simulink library "MCHP_Blockset"  (R2014b)
settings: Solver=ode45  SolverMode=SingleTasking  StartTime=0.0  StopTime=10.0  RelTol=1e-3
InitFcn:
  | disp('MCHP_Blockset_Library_InitFunction');
undefined symbols (not defined in the file): A0, A2, AD0, AVdd, B1, B5, B9, C10, C2, CMP2A, CMP3A, CMP4A, EXTREF1, EXTREF2, gcbh, MaxPer, MCHP_ACC_SAMx_Callback, MCHP_ADC_Callback, MCHP_ADC_HighSpeed_SAR_Callback, MCHP_ADC_HighSpeed_SAR_dsPIC_Callback, MCHP_ADC_SAME5x_Callback, MCHP_AFEC_SAM7x_Callback, MCHP_BUS_I2C_MASTER_callback, MCHP_BUS_SPI_callback, MCHP_C_function_Call_callback, MCHP_CN_Callback, MCHP_COMPARATOR1_callback, MCHP_CompilerOptimisation_Callback, MCHP_DACC_SAMx_Callback, MCHP_Digital_Input_Callback, MCHP_Digital_Output_Read_Callback, MCHP_Digital_Output_Write_Callback, MCHP_Fun, MCHP_HighSpeed_AnalogComparator_Callback, MCHP_IC_Callback, MCHP_IdleTask_Callback, MCHP_Interrupt_Callback, MCHP_Master_Callback, MCHP_MCPWM_Callback, MCHP_MCU_LOAD_Callback, MCHP_MCU_OVERLOAD_Callback, MCHP_MSI_Callback, MCHP_OC_HW_Callback, MCHP_OC_SW_Callback, MCHP_OP_AMP_Callback, MCHP_OrderInOut, MCHP_PDEC_Callback, MCHP_PGA_Callback, MCHP_PWM_Callback, MCHP_PWM_HighSpeed_Override_Callback, MCHP_PWM_HS_FEP_Callback, MCHP_PWM_SAM7x_Callback, MCHP_PWM_SAM7x_Override_Callback, MCHP_QDEC_SAMx_Callback, MCHP_QEI_Callback, MCHP_Scheduler_Options_Callback, MCHP_SECONDARY_CORE_Callback, MCHP_Tasks_State_Callback, MCHP_TCC_PWM_Callback, MCHP_TIMER_Config_Callback ... (+18)
libraries: MCHP_Blockset x2
(part 4 of 9)

== system MCHP_Blockset/BUS I2C ==
  BUS I2C MASTER : S-Function  FunctionName=MCHP_BUS_I2C_MASTER  Parameters=MCHP_BUS_I2C_MASTER_callback(gcbh,'S_INPUT'),MCHP_BUS_I2C_MASTER_callback(gcbh,'S_OUTPUT'),MCHP_BUS_I2C_MASTER_callback(gcbh,'S_INPUT_Size'),MCHP_BUS_I2C_MASTER_callback(gcbh,'S_OUTPUT_Size'),[],SampleTime,MCHP_OrderInOut(gcbh),strcmp(BlockingMode,'on')  EnableBusSupport=off  mask(I2C Driver){I2CRef=1, I2C_IntPriority=5, I2Csequence_txt=Initial-Configuration$     ---     $Start$Write Address:{[0x77]}    % Componnent address$Write Data (x1)  Write:{[0x00]}      % Write a constant$Re-Start$Read Data (x1)  Read:{D2}    % Read a value$Stop, I2Csequence_num=[BFF0000000000000 40E0600000000000 40F86A0000000000 40F866E066594CA2]$[4070000000000000]$[3FF0000000000000 40E0200000000000 40F86A0000000000 40F866E066594CA2]$[4040000000000000 0000000000000000 0000000000000000 405DC00000000000]$[4050000000000000 3FF0000000000000 0000000000000000 0000000000000000]$[4008000000000000 40E0200000000000 40F86A0000000000 40F866E066594CA2]$[4060000000000000 3FF0000000000000]$[4000000000000000 40E0600000000000 40F86A0000000000 40F866E066594CA2], InitialConfigurationNum=0, PIN_SDA_TXT=Dynamic Options, PIN_SCL_TXT=Dynamic Options, S_INPUT=[5  5], S_OUTPUT=[5], S_INPUT_Size=[2  2], S_OUTPUT_Size=[4], BlockingMode=off, SequenceCompleted=off, SampleTime=-1, MCHP_MASTERLINK=Board28PIN_33EP12MC202_I2C_MS5611_V02/Microchip Master, MCHP_PORT={I2C 1 Clock}{SCL1}13:0:B8;{I2C 1 SDA}{SDA1}13:0:B9;, MCHP_USER_INTERRUPTS=, ORDERING=0}
      mask prompts: I2C_IntPriority "Interrupt Priority"; I2Csequence_txt "I2C_Sequence"; I2Csequence_num "I2C_Sequence"; SampleTime "Sample Time"; ORDERING "MCHP_OrderInOut"
      mask init:
      | MCHP_BUS_I2C_MASTER_callback(gcbh,'INITIALISATION');
      settings: CopyFcn=MCHP_BUS_I2C_MASTER_callback(gcbh,'COPY');  DeleteFcn=MCHP_BUS_I2C_MASTER_callback(gcbh,'DELETE');  ModelCloseFcn=MCHP_BUS_I2C_MASTER_callback(gcbh,'MODELCLOSE');  OpenFcn=MCHP_BUS_I2C_MASTER_callback(gcbh,'OPEN');
      mask Display:
      | MCHP_DrawLogo;fprintf(['I2C ' int2str(I2CRef) ' ']);
      | 
      | port_label('output',1,'1/z*D2');

== system MCHP_Blockset/BUS SPI ==
  BUS SPI : S-Function  FunctionName=MCHP_BUS_SPI  Parameters=MCHP_BUS_SPI_callback(gcbh,'S_INPUT'),MCHP_BUS_SPI_callback(gcbh,'S_OUTPUT'),MCHP_BUS_SPI_callback(gcbh,'S_INPUT_Size'),MCHP_BUS_SPI_callback(gcbh,'S_OUTPUT_Size'),[],SampleTime,MCHP_OrderInOut(gcbh),strcmp(BlockingMode,'on')  EnableBusSupport=off  mask(SPI Driver){SPIRef=1, DMA=[0  2  3], SPI_IntPriority=4, SPIsequence_txt=Initial-Configuration$     ---     $Set Port B6 / Pin[42] to 1$Read & Write (x1)  Write:{In}  Read:{out}$Set Port B6 / Pin[42] to 0, SPIsequence_num=[BFF0000000000000 4091B40000000000 0000000000000000 40E0000000000000 411E848000000000 411E848000000000]$[4070000000000000]$[4010000000000000 4036000000000000 3FF0000000000000]$[4008000000000000 3FF0000000000000 3FF0000000000000]$[4010000000000000 4036000000000000 0000000000000000], PIN_SDI_TXT=Dynamic Options, PIN_SDO_TXT=Dynamic Options, PIN_SCK_TXT=Dynamic Options, PIN_SS_TXT=Dynamic Options, S_INPUT=[5  5], S_OUTPUT=[5], S_INPUT_Size=[2  2], S_OUTPUT_Size=[4], BlockingMode=off, SampleTime=-1, MCHP_MASTERLINK=UTester_33EP64MC504_SPI/Microchip Master, MCHP_PORT={SPI 1 input}{SDI1}12:0:A9;{SPI 1 output}{SDO1}12:1:A4;{SPI 1 Clock output}{SCK1}12:1:C3;{SPI 1 PIN output}{SPI1 Pin}12:1:B6;{SPI 1 PIN output}{SPI1 Pin}12:1:B6;, MCHP_USER_INTERRUPTS=, ORDERING=0}
      mask prompts: DMA "DMA [Enabled(0/1) Rx Tx]"; SPI_IntPriority "Interrupt Priority"; SPIsequence_txt "SPI_Sequence"; SPIsequence_num "SPI_Sequence"; SampleTime "Sample Time"; ORDERING "MCHP_OrderInOut"
      mask init:
      | MCHP_BUS_SPI_callback(gcbh,'INITIALISATION');
      settings: CopyFcn=MCHP_BUS_SPI_callback(gcbh,'COPY');  DeleteFcn=MCHP_BUS_SPI_callback(gcbh,'DELETE');  ModelCloseFcn=MCHP_BUS_SPI_callback(gcbh,'MODELCLOSE');  OpenFcn=MCHP_BUS_SPI_callback(gcbh,'OPEN');
      mask Display:
      | MCHP_DrawLogo;fprintf(['SPI ' int2str(SPIRef) ' ']);
      | 
      | port_label('input',1,'In');
      | port_label('output',1,'1/z*out');

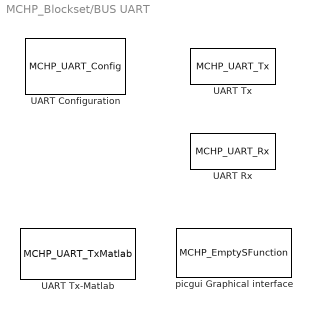
== system MCHP_Blockset/BUS UART ==
  UART Configuration : S-Function  InitFcn=MCHP_UART_Config_Callback(gcbh,'InitFcn');  FunctionName=MCHP_UART_Config  EnableBusSupport=off  mask(Configuration for UART peripheral){UART_REF=1, BAUD_Choice=Dynamic Options, BAUD_Choice_TXT=115200, BAUD_Choice_IR=Dynamic Options, BAUD_Choice_IR_TXT=[], BAUD_Custom=115200, INT_PRIORITY=0, ALT_IO=on, PIN_RX=Dynamic Options, PIN_RX_TXT=Dynamic Options, PIN_TX=Dynamic Options, PIN_TX_TXT=Dynamic Options, MCHP_PORT={UART1  Rx}{U1RX}3:0:P25;{UART1  Tx}{U1TX}3:1:P20;, MCHP_MASTERLINK=0, MCHP_COM_ExtPil=off, TX_IMPLEMENTATION=Circular Buffer, TX_IMPLEMENTATION_default=Circular Buffer, TX_INT_PRIORITY=5, TX_INT_WHEN=is empty, TX_INT_WHEN_default=is empty & last char is sent, TX_CIRCULAR_SIZE=128, TX_DMA_CHANNEL=0   (Lowest Priority), TX_DMA_SIZE=[], TX_TASK_PROTECTION=Delay tasks (default), TX_INTERRUPT_PROTECTION=Do not send on conflict (default), TX_INTERRUPT_PROTECTION_default=Do not send on conflict (default), RX_IMPLEMENTATION=Circular Buffer, RX_IMPLEMENTATION_default=Circular Buffer, RX_INT_PRIORITY=5, RX_INT_WHEN=receive 1 character, RX_CIRCULAR_SIZE=128, RX_DMA_CHANNEL=0, RX_DMA_SIZE=0, DuplexMode=Full duplex (default), PIN_RX_Inv=off, PIN_TX_Inv=off, PIN_RXTX_Inv=off, ParityBit=No parity (default), StopBit=1 stop bit (default), IRDA=off, FlowControl=None, PIN_CTS=Dynamic Options, PIN_CTS_TXT=Dynamic Options, PIN_RTS=Dynamic Options, PIN_RTS_TXT=Dynamic Options, InitSequence_chkbox=off, BAUD_Choice_InitSeq=Dynamic Options, BAUD_Choice_InitSeq_TXT=0, BAUD_Choice_IR_InitSeq=Dynamic Options, BAUD_Choice_IR_InitSeq_TXT=0, BAUD_Custom_InitSeq=0, InitSequence='Hello World'}
      mask prompts: UART_REF "Ref UART"; BAUD_Choice "Current Baud:"; BAUD_Choice_TXT "Baud_Choixe_TXT"; BAUD_Choice_IR "Current Baud:"; BAUD_Custom "Custom Baud: 109306 with -5.12% Error"; INT_PRIORITY "Interrupt Priority"; ALT_IO "Alternative I/O"; PIN_RX "Rx Pin"; PIN_TX "Tx Pin"; TX_IMPLEMENTATION "Implementation"; TX_IMPLEMENTATION_default "Implementation"; TX_INT_PRIORITY "Interrupt Priority"; TX_INT_WHEN "Interrupt when Transmit Buffer"; TX_INT_WHEN_default "Interrupt when Transmit Buffer"; TX_CIRCULAR_SIZE "Circular Buffer size"; TX_DMA_CHANNEL "DMA Channel"; TX_DMA_SIZE "DMA Buffer size"; TX_TASK_PROTECTION "Task intertwined Tx protection"; TX_INTERRUPT_PROTECTION "Asynchronous intertwined Tx protection"; TX_INTERRUPT_PROTECTION_default "Asynchronous intertwined Tx protection"; RX_IMPLEMENTATION "Implementation"; RX_IMPLEMENTATION_default "Implementation"; RX_INT_PRIORITY "Interrupt Priority"; RX_INT_WHEN "Interrupt when Receive Buffer"; RX_CIRCULAR_SIZE "Circular Buffer size"; RX_DMA_CHANNEL "DMA Channel"; RX_DMA_SIZE "DMA Buffer size"; DuplexMode "Duplex"; PIN_RX_Inv "Invert Rx Pin logic (Idle state is low level)"; PIN_TX_Inv "Invert Tx Pin logic (Idle state is low level)"; PIN_RXTX_Inv "Invert Rx & Tx Pin logic (Idle state is low level)"; ParityBit "Parity"; StopBit "Stop bit"; IRDA "IrDA Mode"; FlowControl "Hardware Flow Control"; PIN_CTS "CTS Pin (input)"; PIN_RTS "RTS Pin (output)"; InitSequence_chkbox "Send an Initialisation sequence on the UART"; BAUD_Choice_InitSeq "Baud for initialisation sequence:"; BAUD_Choice_InitSeq_TXT "Baud_Choixe_TXT"; BAUD_Choice_IR_InitSeq "Baud for initialisation sequence:"; BAUD_Choice_IR_InitSeq_TXT "Baud_Choice_IR_TXT"; BAUD_Custom_InitSeq "Custom Baud: 109306 with -5.12% Error"; InitSequence "Initialisaiton sequence to send (String or vector)"
      mask init:
      | MCHP_UART_Config_Callback(gcbh,'INITIALISATION');
      settings: CopyFcn=MCHP_UART_Config_Callback(gcbh,'CopyFcn');  PreSaveFcn=MCHP_Fun.PreSaveFcn_DynamicOptions(gcbh);  OpenFcn=MCHP_UART_Config_Callback(gcbh,'OPEN');
      mask TypeOptions UART_REF: 1 | 2 | 3 | 4 | 5 | 6 | 7 | 8 | 9 | USART 0 | USART 1 | USART 2 | USART 3 | USART 4 | USART 5 | USART 6 | USART 7 | USART 8 | ----------- | UART 0 | UART 1 | UART 2 | UART 3 | UART 4 | UART 5 | UART 6 | UART 7 | UART 8 | --SAMx5----- | SERCOM USART 0 | SERCOM USART 1 | SERCOM USART 2 | SERCOM USART 3 | SERCOM USART 4 | SERCOM USART 5 | SERCOM USART 6 | SERCOM USART 7 | SERCOM USART 8 | SERCOM USART 9
      mask Callback UART_REF: MCHP_UART_Config_Callback(gcbh,'UART_REF');
      mask TypeOptions BAUD_Choice: Dynamic Options
      mask Callback BAUD_Choice: MCHP_UART_Config_Callback(gcbh,'BAUD_Choice');
      mask TypeOptions BAUD_Choice_IR: Dynamic Options
      mask Callback BAUD_Choice_IR: MCHP_UART_Config_Callback(gcbh,'BAUD_Choice_IR');
      mask Callback BAUD_Choice_IR_TXT: % This field is not used
      mask Callback BAUD_Custom: MCHP_UART_Config_Callback(gcbh,'BAUD_Custom');
      mask TypeOptions INT_PRIORITY: 0 | 1 | 2 | 3 | 4 | 5 | 6 | 7
      mask TypeOptions PIN_RX: Dynamic Options
      mask TypeOptions PIN_TX: Dynamic Options
      mask TypeOptions TX_IMPLEMENTATION: Do not implement Tx | Simplest (1 bytes internal buffer only) | Simplest (4 bytes internal buffer only) | Simplest (8 bytes internal buffer only) | Circular Buffer | DMA Ping-Pong Mode | DMA single Buffer (Possible data loss)
      mask Callback TX_IMPLEMENTATION: MCHP_UART_Config_Callback(gcbh,'TX_IMPLEMENTATION');
      mask TypeOptions TX_IMPLEMENTATION_default: Circular Buffer
      mask TypeOptions TX_INT_PRIORITY: 0 | 1 | 2 | 3 | 4 | 5 | 6 | 7
      mask TypeOptions TX_INT_WHEN: is empty | is empty & last char is sent | has one empty space
      mask TypeOptions TX_INT_WHEN_default: is empty & last char is sent
      mask TypeOptions TX_CIRCULAR_SIZE: 4 | 8 | 16 | 32 | 64 | 128 | 256 | 512 | 1024 | 2048 | 4096 | 8192 | 16384 | 32768
      mask TypeOptions TX_DMA_CHANNEL: 0 | 0   (Lowest Priority) | 1 | 2 | 3 | 4 | 5 | 6 | 7 | 8 | 9 | 10 | 11 | 12 | 13 | 14 | 15 | 16 | 17 | 18 | 19 | 20 | 21 | 22 | 23
      mask TypeOptions TX_TASK_PROTECTION: Delay tasks (default) | Do not send on conflict | no protection
      mask Callback TX_TASK_PROTECTION: MCHP_UART_Config_Callback(gcbh,'TX_TASK_PROTECTION');
      mask TypeOptions TX_INTERRUPT_PROTECTION: Do not send on conflict (default) | Delay all interrupts | no protection
      mask TypeOptions TX_INTERRUPT_PROTECTION_default: Do not send on conflict (default)
      mask TypeOptions RX_IMPLEMENTATION: Do not implement Rx | Simplest (1 bytes internal buffer only) | Simplest (4 bytes internal buffer only) | Simplest (8 bytes internal buffer only) | Circular Buffer | DMA Ping-Pong | DMA Single Buffer (possible data loss)
      mask Callback RX_IMPLEMENTATION: MCHP_UART_Config_Callback(gcbh,'RX_IMPLEMENTATION');
      mask TypeOptions RX_IMPLEMENTATION_default: Circular Buffer
      mask TypeOptions RX_INT_PRIORITY: 1 | 2 | 3 | 4 | 5 | 6 | 7
      mask TypeOptions RX_INT_WHEN: is full (contains 4 data characters) | is 3/4 fulll (contains 3 data characters) | receive 1 character
      mask TypeOptions RX_CIRCULAR_SIZE: 4 | 8 | 16 | 32 | 64 | 128 | 256 | 512 | 1024 | 2048 | 4096 | 8192 | 16384 | 32768
      mask TypeOptions RX_DMA_CHANNEL: 0 | 0   (Lowest Priority) | 1 | 2 | 3 | 4 | 5 | 6 | 7 | 8 | 9 | 10 | 11 | 12 | 13 | 14 | 15 | 16 | 17 | 18 | 19 | 20 | 21 | 22 | 23
      mask TypeOptions DuplexMode: Full duplex (default) | Half duplex for one wire Rx-Tx specific case
      mask Callback DuplexMode: MCHP_UART_Config_Callback(gcbh,'DuplexMode');
      mask TypeOptions ParityBit: No parity (default) | Even | Odd | Space (force to 0) | Mark (force to 1) | Multidrop
      mask TypeOptions StopBit: 1 stop bit (default) | 1.5 stop bits | 2 stop bits
      mask Callback IRDA: MCHP_UART_Config_Callback(gcbh,'IRDA');
      mask TypeOptions FlowControl: None | RTS / CTS
      mask Callback FlowControl: MCHP_UART_Config_Callback(gcbh,'FlowControl');
      mask TypeOptions PIN_CTS: Dynamic Options
      mask TypeOptions PIN_RTS: Dynamic Options
      mask Callback InitSequence_chkbox: MCHP_UART_Config_Callback(gcbh,'InitSequence_chkbox');
      mask TypeOptions BAUD_Choice_InitSeq: Dynamic Options
      mask Callback BAUD_Choice_InitSeq: MCHP_UART_Config_Callback(gcbh,'BAUD_Choice_InitSeq');
      mask TypeOptions BAUD_Choice_IR_InitSeq: Dynamic Options
      mask Callback BAUD_Choice_IR_InitSeq: MCHP_UART_Config_Callback(gcbh,'BAUD_Choice_IR_InitSeq');
      mask Callback BAUD_Custom_InitSeq: MCHP_UART_Config_Callback(gcbh,'BAUD_Custom_InitSeq');
      mask Display:
      | MCHP_DrawLogo;
      | disp('UART Config');
  UART Rx : S-Function  FunctionName=MCHP_UART_Rx  Parameters=SampleTime,strcmp(Flag_Out,'on'),S_Rx_Size,MCHP_OrderInOut(gcbh)  EnableBusSupport=off  mask(UART Rx Input Driver){UART_REF=1, Flag_Out=off, Rx_Size_popup=User defined, Rx_Size=1, S_Rx_Size=1, Split=Read all received char, SplitChar=10, OutputDefault_popup=Fill-in output vector with specified value, OutputDefault=-1, ORDERING=None, SampleTime=-1, MCHP_MASTERLINK=UTestBoard_33FJ256GP710A_2/Microchip Master, MCHP_COMPILED_INFO=0}
      mask prompts: UART_REF "UART Ref"; Flag_Out "Output Number of char read"; Rx_Size_popup "Vector Output size"; Rx_Size "Vector Output size (i.e. try to read n char)"; SplitChar "Stop reading on character: (split)"; OutputDefault_popup "Fill-in output vector when not full:"; OutputDefault "Output Vector not full: fill in with value: (-1 repeat last char, -2: do nothing)"; ORDERING "Block execution ordering"; SampleTime "Sample Time"
      mask help:
      | Receive data (8 bits datatype) through the UART.use >>picgui at the Matlab prompt in "raw" mode to send/receive data with matlab.
      |
      | UART Ports: [ Rx  Tx  ]
      | UART 1:         [ F2  F3 ]
      | UART 2:         [ F4  F5 ]
      |
      | UART 2 is configured at:   115200         [-0.04%]
      mask init:
      | MCHP_UART_Rx_Callback(gcbh,'INITIALISATION');
      settings: OpenFcn=MCHP_UART_Rx_Callback(gcbh,'OPEN');
      mask TypeOptions UART_REF: 1 | 2 | 3 | 4 | 5 | 6 | 7 | 8 | 9 | USART 0 | USART 1 | USART 2 | USART 3 | USART 4 | USART 5 | USART 6 | USART 7 | USART 8 | ----------- | UART 0 | UART 1 | UART 2 | UART 3 | UART 4 | UART 5 | UART 6 | UART 7 | UART 8
      mask Callback UART_REF: MCHP_UART_Rx_Callback(gcbh,'UART_REF');
      mask TypeOptions Rx_Size_popup: User defined | Inherited via back propagation | Inherited via internal rule
      mask Callback Rx_Size_popup: MCHP_UART_Rx_Callback(gcbh,'Rx_Size_popup');
      mask Callback Rx_Size: MCHP_UART_Rx_Callback(gcbh,'Rx_Size');
      mask TypeOptions Split: Read all received char | Stop reading when one specified char is detected
      mask Callback Split: MCHP_UART_Rx_Callback(gcbh,'Split');
      mask TypeOptions OutputDefault_popup: Fill-in output vector with specified value | Add one trailing 0 | do nothing (end of output vector will be undefined)
      mask Callback OutputDefault_popup: MCHP_UART_Rx_Callback(gcbh,'OutputDefault_popup');
      mask TypeOptions ORDERING: None | Input | Output | Input & Output
      mask Display: MCHP_DrawLogo;fprintf('UART 1\nRx');port_label('output',1,'Rx' );
  UART Tx : S-Function  FunctionName=MCHP_UART_Tx  Parameters=SampleTime,MCHP_OrderInOut(gcbh),NSend_Input,NSend_Output  EnableBusSupport=off  mask(UART Tx Output Driver){UART_REF=1, ORDERING=None, AllOrNothing=off, SampleTime=-1, MCHP_MASTERLINK=0, NSend_Input=off, UART_String=off, NSend_Output=off}
      mask prompts: UART_REF "UART Ref"; ORDERING "Block execution ordering"; AllOrNothing "UART Overflow: Send all or nothing"; SampleTime "Sample Time"; NSend_Input "Send first N bytes from the vector input with N a block input"; UART_String "With vector input, do not send values following the first 0 (string like)"; NSend_Output "Number of byte sent is a block output"
      mask init:
      | MCHP_UART_Tx_Callback(gcbh,'INITIALISATION');
      settings: OpenFcn=MCHP_UART_Tx_Callback(gcbh,'OPEN');
      mask TypeOptions UART_REF: 0 | 1 | 2 | 3 | 4 | 5 | 6 | 7 | 8 | 9 | USART 0 | USART 1 | USART 2 | USART 3 | USART 4 | USART 5 | USART 6 | USART 7 | USART 8 | ----------- | UART 0 | UART 1 | UART 2 | UART 3 | UART 4 | UART 5 | UART 6 | UART 7 | UART 8
      mask Callback UART_REF: MCHP_UART_Tx_Callback(gcbh,'UART_REF');
      mask TypeOptions ORDERING: None | Input | Output | Input & Output
      mask Display: MCHP_DrawLogo;fprintf('UART 1\nTx');port_label('input',1,'Tx' );
  UART Tx-Matlab : S-Function  FunctionName=MCHP_UART_TxMatlab  Parameters=SampleTime,MCHP_UART_TxMatlab_Callback(gcbh,'S_INPUT')  EnableBusSupport=off  mask(Higl Level UART protocol){UART_REF=1, CHANNELS=[1 2 ], AllOrNothing=off, SampleTime=-1, MCHP_MASTERLINK=MCHP_Blockset/System Configuration/Microchip Master, MCHP_COMPILED_INFO=CompiledSampleTime= [0.001   0 ];CompiledPortDataTypes=[  5   5   5   5   5   3 ];}
      mask prompts: UART_REF "UART Ref"; CHANNELS "Channels (Matlab Columns)"; AllOrNothing "UART Overflow: Send all or nothing"; SampleTime "Sample Time"
      mask init:
      | MCHP_UART_TxMatlab_Callback(gcbh,'INITIALISATION');
      settings: OpenFcn=MCHP_UART_TxMatlab_Callback(gcbh,'OPEN');
      mask TypeOptions UART_REF: 0 | 1 | 2 | 3 | 4 | 5 | 6 | 7 | 8 | 9 | USART 0 | USART 1 | USART 2 | USART 3 | USART 4 | USART 5 | USART 6 | USART 7 | USART 8 | ----------- | UART 0 | UART 1 | UART 2 | UART 3 | UART 4 | UART 5 | UART 6 | UART 7 | UART 8
      mask Callback UART_REF: MCHP_UART_TxMatlab_Callback(gcbh,'UART_REF');
      mask Callback CHANNELS: MCHP_UART_TxMatlab_Callback(gcbh,'INITIALISATION');
      mask Display: MCHP_DrawLogo;fprintf('UART 1\n>Matlab');port_label('input',1,'CH 1 ' );port_label('input',2,'CH 2 ' );
  picgui Graphical interface : S-Function  FunctionName=MCHP_EmptySFunction  EnableBusSupport=off  mask{Nothing=0}
      settings: OpenFcn=picgui;
      mask Display:
      | MCHP_DrawLogo;
      | color('black');
      | disp('Interface\nTx-Matlab\n>>picgui')

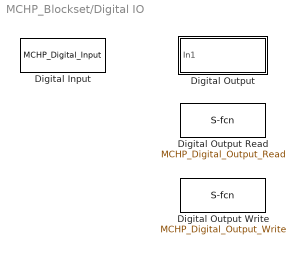
== system MCHP_Blockset/Digital IO ==
  Digital Input : S-Function  FunctionName=MCHP_Digital_Input  Parameters=SampleTime,[],MCHP_Digital_Input_Callback(gcb,'S_OUTPUT'),MCHP_OrderInOut(gcbh)  EnableBusSupport=off  mask(Input driver for Digital Input Pins){PORT=Dynamic Options, PORT_TXT=A0, PIN=[0], PACK=off, SIMULTANEOUS=off, ORDERING=None, SampleTime=-1, MCHP_PORT={Digital In}2:0:A0;, MCHP_MASTERLINK=0}
      mask prompts: PORT_TXT "Port TXT"; PIN "Pins : [ 0 : 4 ]"; PACK "set output as one uint16"; SIMULTANEOUS "Exact simultaneous sample"; ORDERING "Block execution ordering"; SampleTime "Sample Time"
      mask help:
      | Selected pin(s) are configured as a digital input.
      |
      | When the block output is defined as one uint16, user should
      | take into account only bits corresponding to pins selected.
      mask init:
      | MCHP_Digital_Input_Callback(gcb,'INITIALISATION');
      settings: PreSaveFcn=MCHP_Fun.PreSaveFcn_DynamicOptions(gcbh);  OpenFcn=MCHP_Digital_Input_Callback(gcb,'OPEN');
      mask TypeOptions PORT: Dynamic Options
      mask Callback PORT: MCHP_Fun.BlockUpdate(gcbh);
      mask Callback PIN: MCHP_Fun.BlockUpdate(gcbh);
      mask Callback PACK: MCHP_Fun.BlockUpdate(gcbh);
      mask Callback SIMULTANEOUS: %MCHP_Fun.BlockUpdate(gcbh);
      mask TypeOptions ORDERING: None | Input | Output | Input & Output
      mask Display:
      | MCHP_DrawLogo;
      | fprintf('Digital\nInput');
      | port_label('output',1,'A0');
  Digital Output : Subsystem  mask{PORT=Dynamic Options, PORT_TXT=A   [ 0  1  2  3  4  5  6  7  9  10  14  15 ], PIN=[0], PACK=off, SIMULTANEOUS=off, READPREVIOUS=off, ORDERING=None, SampleTime=-1, MCHP_PORT={Digital Out}{DOU}1:1:A0;{Digital Out}{DOU}1:1:A1;{Digital Out}{DOU}1:1:A2;, MCHP_MASTERLINK=UTester_33EP512MU810_NewDigitOutBlock/Microchip Master}
      mask prompts: PORT_TXT "Port TXT"; PIN "PORT A Indexes within [ 0  1  2  3  4  5  6  7  9  10  14  15 ]"; PACK "set input as one uint16"; SIMULTANEOUS "Exact simulatneous update"; READPREVIOUS "Read previous value written (1/z delay)"; ORDERING "Block execution ordering"; SampleTime "Sample Time"
      mask init:
      | MCHP_Digital_Output_Callback(gcb,'INITIALISATION');
      settings: PreSaveFcn=MCHP_Fun.PreSaveFcn_DynamicOptions(gcbh);  OpenFcn=MCHP_Digital_Output_Callback(gcb,'OPEN');
      mask TypeOptions PORT: Dynamic Options
      mask Callback PORT: MCHP_Fun.BlockUpdate(gcbh);
      mask Callback PIN: MCHP_Fun.BlockUpdate(gcbh);
      mask Callback PACK: MCHP_Fun.BlockUpdate(gcbh);
      mask Callback SIMULTANEOUS: MCHP_Fun.BlockUpdate(gcbh);
      mask Callback READPREVIOUS: MCHP_Fun.BlockUpdate(gcbh);
      mask TypeOptions ORDERING: None | Input | Output | Input & Output
      mask Callback ORDERING: MCHP_Fun.BlockUpdate(gcbh);
      mask Display:
      | MCHP_DrawLogo;fprintf('Digital\nOutput')
      | port_label('input',1,'A0');
  Digital Output Read : S-Function  FunctionName=MCHP_Digital_Output_Read  Parameters=SampleTime,MCHP_Digital_Output_Read_Callback(gcb,'S_INPUT'),MCHP_Digital_Output_Read_Callback(gcb,'S_OUTPUT'),MCHP_OrderInOut(gcbh)  EnableBusSupport=off  mask(Output driver for Digital Output Pins){PORT=Dynamic Options, PORT_TXT=A   [ 0  1  2  3  4  5  6  7  9  10  14  15 ], PIN=0, PACK=off, SIMULTANEOUS=off, READPREVIOUS=off, ORDERING=None, SampleTime=.1, MCHP_PORT={Digital Out}{DOU}1:1:A0;, MCHP_MASTERLINK=UTester_33EP512MU810_NewDigitOutBlock/Microchip Master}
      mask prompts: PORT_TXT "Port TXT"; PIN "PORT A Indexes within [ 0  1  2  3  4  5  6  7  9  10  14  15 ]"; PACK "set output as one uint16"; SIMULTANEOUS "Exact simultaneous update"; READPREVIOUS "Read previous value written (1/z delay)"; ORDERING "Block execution ordering"; SampleTime "Sample Time"
      mask help:
      | Selected pin(s) are configured as a digital output.
      |
      | When the block input is defined as one uint16, the value
      | is beeing used as is without masks.
      | This behaviour might affect others pins from the same port
      | provided they are configured as digital output as well.
      mask init:
      | MCHP_Digital_Output_Read_Callback(gcb,'INITIALISATION');
      settings: PreSaveFcn=MCHP_Fun.PreSaveFcn_DynamicOptions(gcbh);  OpenFcn=MCHP_Digital_Output_Read_Callback(gcb,'OPEN');
      mask TypeOptions PORT: Dynamic Options
      mask Callback PORT: MCHP_Fun.BlockUpdate(gcbh);
      mask Callback PIN: MCHP_Fun.BlockUpdate(gcbh);
      mask Callback PACK: MCHP_Fun.BlockUpdate(gcbh);
      mask Callback SIMULTANEOUS: %MCHP_Digital_Output_Read_Callback(gcb,'SIMULTANEOUS');
      mask TypeOptions ORDERING: None | Input | Output | Input & Output
      mask Display:
      | MCHP_DrawLogo;fprintf('Digital\nOutput\nRead')
      | port_label('output',1,'A0');
  Digital Output Write : S-Function  FunctionName=MCHP_Digital_Output_Write  Parameters=SampleTime,MCHP_Digital_Output_Write_Callback(gcb,'S_INPUT'),MCHP_Digital_Output_Write_Callback(gcb,'S_OUTPUT'),MCHP_OrderInOut(gcbh)  EnableBusSupport=off  mask(Output driver for Digital Output Pins){PORT=Dynamic Options, PORT_TXT=A   [ 0  1  2  3  4  5  6  7  9  10  14  15 ], PIN=0, PACK=off, SIMULTANEOUS=off, ORDERING=None, SampleTime=-1, MCHP_PORT={Digital Out}{DOU}1:1:A0;, MCHP_MASTERLINK=UTester_33EP512MU810_NewDigitOutBlock/Microchip Master}
      mask prompts: PORT_TXT "Port TXT"; PIN "PORT A Indexes within [ 0  1  2  3  4  5  6  7  9  10  14  15 ]"; PACK "set input as one uint16"; SIMULTANEOUS "Exact simultaneous update"; ORDERING "Block execution ordering"; SampleTime "Sample Time"
      mask help:
      | Selected pin(s) are configured as a digital output.
      |
      | When the block input is defined as one uint16, the value
      | is beeing used as is without masks.
      | This behaviour might affect others pins from the same port
      | provided they are configured as digital output as well.
      mask init:
      | MCHP_Digital_Output_Write_Callback(gcb,'INITIALISATION');
      settings: PreSaveFcn=MCHP_Fun.PreSaveFcn_DynamicOptions(gcbh);  OpenFcn=MCHP_Digital_Output_Write_Callback(gcb,'OPEN');
      mask TypeOptions PORT: Dynamic Options
      mask Callback PORT: MCHP_Fun.BlockUpdate(gcbh);
      mask Callback PIN: MCHP_Fun.BlockUpdate(gcbh);
      mask Callback PACK: MCHP_Fun.BlockUpdate(gcbh);
      mask Callback SIMULTANEOUS: %MCHP_Digital_Output_Write_Callback(gcb,'SIMULTANEOUS');
      mask TypeOptions ORDERING: None | Input | Output | Input & Output
      mask Display:
      | MCHP_DrawLogo;fprintf('Digital\nOutput\nWrite')
      | port_label('input',1,'A0');

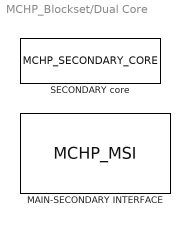
== system MCHP_Blockset/Dual Core ==
  MAIN-SECONDARY INTERFACE : S-Function  InitFcn=MCHP_MSI_Callback(gcb,'InitFcn');  FunctionName=MCHP_MSI  Parameters=MCHP_MSI_Callback(gcbh,'S_INPUT'),MCHP_MSI_Callback(gcbh,'S_OUTPUT'),MCHP_MSI_Callback(gcbh,'S_INPUT_Size'),MCHP_MSI_Callback(gcbh,'S_OUTPUT_Size'),MCHP_MSI_Callback(gcbh,'S_ListCustomDatatype'),SampleTime,0  EnableBusSupport=off  mask(Main core / Secondary core data INTERFACE){direction=send to main core, Offset=5, protocol=use protocol A, NData=3, Data1=unsigned int16, Data2=unsigned int8, Data3=single, Data4=signed int16, Data5=signed int16, Data6=signed int16, Data7=signed int16, Data8=signed int16, Data9=signed int16, Data10=signed int16, Data11=signed int16, Data12=signed int16, Data13=signed int16, Data14=signed int16, Data15=signed int16, Data16=signed int16, Data17=signed int16, Data18=signed int16, Data19=signed int16, Data20=signed int16, Data21=signed int16, Data22=signed int16, Data23=signed int16, Data24=signed int16, Data25=signed int16, Data26=signed int16, Data27=signed int16, Data28=signed int16, Data29=signed int16, Data30=signed int16, Data31=signed int16, Data32=signed int16, info=0, MCHP_MASTERLINK=dsPIC33CH512MP508_MSI_Master/Microchip Master1, SampleTime=-1}
      mask prompts: Offset "Start from Maibox"; protocol "Synchronisation"; NData "Number of data"; Data1 "Data 1"; Data2 "Data 2"; Data3 "Data 3"; Data4 "Data 4"; Data5 "Data 5"; Data6 "Data 6"; Data7 "Data 7"; Data8 "Data 8"; Data9 "Data 9"; Data10 "Data 10"; Data11 "Data 11"; Data12 "Data 12"; Data13 "Data 13"; Data14 "Data 14"; Data15 "Data 15"; Data16 "Data 16"; Data17 "Data 17"; Data18 "Data 18"; Data19 "Data 19"; Data20 "Data 20"; Data21 "Data 21"; Data22 "Data 22"; Data23 "Data 23"; Data24 "Data 24"; Data25 "Data 25"; Data26 "Data 26"; Data27 "Data 27"; Data28 "Data 28"; Data29 "Data 29"; Data30 "Data 30"; Data31 "Data 31"; Data32 "Data 32"; SampleTime "Sample Time"
      mask help:
      | Main and Secondary core data exchange. Sender update data ONLY when previous data have been read by the Receiver.
      |
      | Main and Secondary Interface (MSI) blocks must have the same configuration. Drag & Drop block from Main to Secondary to ensure consistent setting.
      | Mailboxes mechanism is configured depending on settings. When multiple block are used to sent different data at different rate, use the mailbox offset to prevent one mailbox to get re-used.
      | The MSI block with a given setting can be duplicated within a model with a modified sampling time.
      mask init:
      | MCHP_MSI_Callback(gcbh,'INITIALISATION');
      settings: CopyFcn=MCHP_Fun.BlockUpdate(gcbh);  DeleteFcn=MCHP_MSI_Callback(gcbh,'DeleteFcn')  OpenFcn=MCHP_MSI_Callback(gcb,'OPEN');
      mask TypeOptions direction: send to main core | receive from main core | send to secondary core | receive from secondary core
      mask TypeOptions Offset: 0 | 1 | 2 | 3 | 4 | 5 | 6 | 7 | 8 | 9 | 10 | 11 | 12 | 13 | 14 | 15
      mask TypeOptions protocol: use protocol A | use protocol B | use protocol C | use protocol D | use protocol E | use protocol F | use protocol G | use protocol H
      mask TypeOptions NData: 1 | 2 | 3 | 4 | 5 | 6 | 7 | 8 | 9 | 10 | 11 | 12 | 13 | 14 | 15 | 16 | 17 | 18 | 19 | 20 | 21 | 22 | 23 | 24 | 25 | 26 | 27 | 28 | 29 | 30 | 31 | 32
      mask Callback NData: MCHP_MSI_Callback(gcbh,'UpdateGUI');
      mask TypeOptions Data1: unsigned int8 | unsigned int16 | unsigned in32 | --- | signed int8 | signed int16 | signed int32 | ---- | single | double
      mask TypeOptions Data2: unsigned int8 | unsigned int16 | unsigned in32 | --- | signed int8 | signed int16 | signed int32 | ---- | single | double
      mask TypeOptions Data3: unsigned int8 | unsigned int16 | unsigned in32 | --- | signed int8 | signed int16 | signed int32 | ---- | single | double
      mask TypeOptions Data4: unsigned int8 | unsigned int16 | unsigned in32 | --- | signed int8 | signed int16 | signed int32 | ---- | single | double
      mask TypeOptions Data5: unsigned int8 | unsigned int16 | unsigned in32 | --- | signed int8 | signed int16 | signed int32 | ---- | single | double
      mask TypeOptions Data6: unsigned int8 | unsigned int16 | unsigned in32 | --- | signed int8 | signed int16 | signed int32 | ---- | single | double
      mask TypeOptions Data7: unsigned int8 | unsigned int16 | unsigned in32 | --- | signed int8 | signed int16 | signed int32 | ---- | single | double
      mask TypeOptions Data8: unsigned int8 | unsigned int16 | unsigned in32 | --- | signed int8 | signed int16 | signed int32 | ---- | single | double
      mask TypeOptions Data9: unsigned int8 | unsigned int16 | unsigned in32 | --- | signed int8 | signed int16 | signed int32 | ---- | single | double
      mask TypeOptions Data10: unsigned int8 | unsigned int16 | unsigned in32 | --- | signed int8 | signed int16 | signed int32 | ---- | single | double
      mask TypeOptions Data11: unsigned int8 | unsigned int16 | unsigned in32 | --- | signed int8 | signed int16 | signed int32 | ---- | single | double
      mask TypeOptions Data12: unsigned int8 | unsigned int16 | unsigned in32 | --- | signed int8 | signed int16 | signed int32 | ---- | single | double
      mask TypeOptions Data13: unsigned int8 | unsigned int16 | unsigned in32 | --- | signed int8 | signed int16 | signed int32 | ---- | single | double
      mask TypeOptions Data14: unsigned int8 | unsigned int16 | unsigned in32 | --- | signed int8 | signed int16 | signed int32 | ---- | single | double
      mask TypeOptions Data15: unsigned int8 | unsigned int16 | unsigned in32 | --- | signed int8 | signed int16 | signed int32 | ---- | single | double
      mask TypeOptions Data16: unsigned int8 | unsigned int16 | unsigned in32 | --- | signed int8 | signed int16 | signed int32 | ---- | single | double
      mask TypeOptions Data17: unsigned int8 | unsigned int16 | unsigned in32 | --- | signed int8 | signed int16 | signed int32 | ---- | single | double
      mask TypeOptions Data18: unsigned int8 | unsigned int16 | unsigned in32 | --- | signed int8 | signed int16 | signed int32 | ---- | single | double
      mask TypeOptions Data19: unsigned int8 | unsigned int16 | unsigned in32 | --- | signed int8 | signed int16 | signed int32 | ---- | single | double
      mask TypeOptions Data20: unsigned int8 | unsigned int16 | unsigned in32 | --- | signed int8 | signed int16 | signed int32 | ---- | single | double
      mask TypeOptions Data21: unsigned int8 | unsigned int16 | unsigned in32 | --- | signed int8 | signed int16 | signed int32 | ---- | single | double
      mask TypeOptions Data22: unsigned int8 | unsigned int16 | unsigned in32 | --- | signed int8 | signed int16 | signed int32 | ---- | single | double
      mask TypeOptions Data23: unsigned int8 | unsigned int16 | unsigned in32 | --- | signed int8 | signed int16 | signed int32 | ---- | single | double
      mask TypeOptions Data24: unsigned int8 | unsigned int16 | unsigned in32 | --- | signed int8 | signed int16 | signed int32 | ---- | single | double
      mask TypeOptions Data25: unsigned int8 | unsigned int16 | unsigned in32 | --- | signed int8 | signed int16 | signed int32 | ---- | single | double
      mask TypeOptions Data26: unsigned int8 | unsigned int16 | unsigned in32 | --- | signed int8 | signed int16 | signed int32 | ---- | single | double
      mask TypeOptions Data27: unsigned int8 | unsigned int16 | unsigned in32 | --- | signed int8 | signed int16 | signed int32 | ---- | single | double
      mask TypeOptions Data28: unsigned int8 | unsigned int16 | unsigned in32 | --- | signed int8 | signed int16 | signed int32 | ---- | single | double
      mask TypeOptions Data29: unsigned int8 | unsigned int16 | unsigned in32 | --- | signed int8 | signed int16 | signed int32 | ---- | single | double
      mask TypeOptions Data30: unsigned int8 | unsigned int16 | unsigned in32 | --- | signed int8 | signed int16 | signed int32 | ---- | single | double
      mask TypeOptions Data31: unsigned int8 | unsigned int16 | unsigned in32 | --- | signed int8 | signed int16 | signed int32 | ---- | single | double
      mask TypeOptions Data32: unsigned int8 | unsigned int16 | unsigned in32 | --- | signed int8 | signed int16 | signed int32 | ---- | single | double
      mask Display:
      | MCHP_DrawLogo;fprintf('MSI\nto / from');
      | port_label('input', 1 ,' A1 ');
      | port_label('input', 2 ,' A2 ');
      | port_label('output', 1 ,' A1 ');
      | port_label('output', 2 ,' A2 ');
  SECONDARY core : S-Function  InitFcn=MCHP_SECONDARY_CORE_Callback(gcb,'InitFcn');  FunctionName=MCHP_SECONDARY_CORE  Parameters=[],[],[],[],[],-1,0  EnableBusSupport=off  mask(Select Secondary core Image){SLAVE_sFile=dsPIC33CH512MP508_MSI_Slave.X\slave1_image\slave1_image.s, SLAVE_sFile_Save=C:\M91449\MCHP_Blockset\Developpements\2019_08_dsPIC_CH_DualCore\dsPIC33CH512MP508_MSI_Slave.X\slave1_image\slave1_image.s, SLAVE_sFile_Save_relative=\dsPIC33CH512MP508_MSI_Slave.X\slave1_image\slave1_image.s, MCHP_MASTERLINK=dsPIC33CH512MP508_MSI_Master/Microchip Master1}
      mask prompts: SLAVE_sFile "SECONDARY core image path"; SLAVE_sFile_Save "SECONDARY core image path"; SLAVE_sFile_Save_relative "SECONDARY core image path relative"
      mask help:
      | With Dual Core chip, two simulink model are to be used. One for the Main Core, one for the Secondary core.
      | This block added to the Main core simulink model select the secondary core image to be linked with.
      | The secondary core image is the .s file which might be generated by a dedicated Simulink model set with the Secondary core (ending with S1).
      |
      | Output pin must be driven by one core exclusively. Input pins can be used by both core simultaneously.
      mask init:
      | MCHP_SECONDARY_CORE_Callback(gcbh,'INITIALISATION');
      settings: CopyFcn=MCHP_SECONDARY_CORE_Callback(gcb,'COPY');  DeleteFcn=MCHP_SECONDARY_CORE_Callback(gcbh,'DeleteFcn')  OpenFcn=MCHP_SECONDARY_CORE_Callback(gcb,'OPEN');
      mask TypeOptions SLAVE_sFile: None | dsPIC33CH512MP508_MSI_Slave.X\slave1_image\slave1_image.s | Select slave image
      mask Callback SLAVE_sFile: MCHP_Fun.BlockUpdate(gcbh);
